simulink model "mazeSolving"  (R2023a)
settings: Solver=FixedStepDiscrete  StartTime=0.0  StopTime=120  FixedStep=0.01  RelTol=1e-3
values from neighbouring files (symbols this model uses):
  mapForSim =     [localisaton_obstacle_map.mat]
undefined symbols (not defined in the file or in its folder): axleLength, DiscIntNeverNeededParam, lineLength, wheelR
libraries: mobileRoboticsTrainingLib x2
settings Model: Creator=Boitumelo  LastModifiedBy=Nicola
settings DebuggingCC: UnconnectedInputMsg=warning  UnconnectedOutputMsg=warning  UnconnectedLineMsg=warning
settings ModelReferenceCC: EnableRefExpFcnMdlSchedulingChecks=on
settings RTWCC: DLArmComputeVersion=19.05

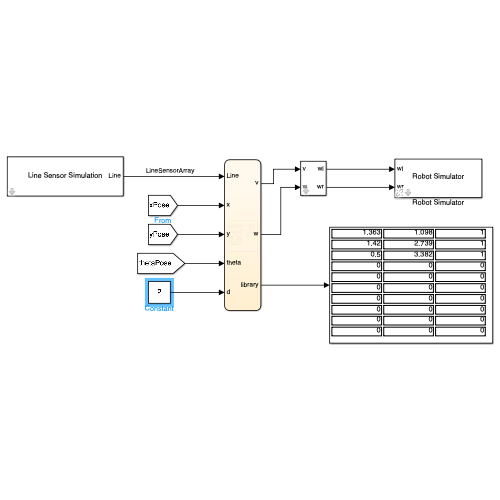
[thumbnail: Simulink's stored preview of the top-level diagram]
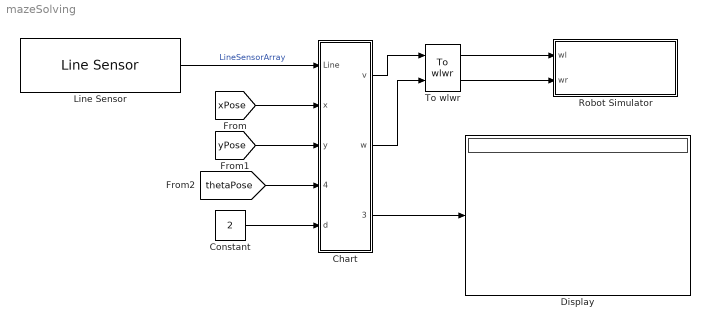
== system mazeSolving ==
  Chart : Stateflow chart  TreatAsAtomicUnit=on
      settings: PortSchema="{\"entries\":[{\"content\":{\"sides\":[{\"content\":{\"connectorIds\":[\"In1\",\"In2\",\"In3\",\"In4\",\"In5\"]},\"type\":\"ConnectorPlacement.EquallySpacedRectSide\",\"uuid\":\"117de8c6-9f64-465b-9576-500dc720da7e\"},{\"content\":{\"connectorIds\":[\"Out2\",\"Out1\",\"Out3\"],\"side\":\"RIGHT\"},\"type\":\"ConnectorPlacement.EquallySpacedRectSide\",\"uuid\":\"fddceec0-8182-4b0d-b09c-ad052d506c18\"},{\"content\":{\"side\":\"TOP\"},\"type\":\"ConnectorPlacement.EquallySpacedRectSide\",\"uuid\":\"0cbecf6e-5fd1-4495-a604-566e504879ee\"}]},\"type\":\"ConnectorPlacement.EquallySpacedConnector\",\"uuid\":\"83bd2747-f15a-41a4-a0f3-2474611a0dc7\"}],\"packageUris\":[\"http://schema.mathworks.com/mf0/Connector/R2020b\"],\"version\":\"1.0\"}"
  Constant : Constant  Value=2
  Display : Display
  Line Sensor : mobileRoboticsTrainingLib/Line Sensor  mapVariable=mapForSim  envVal=1  lineVal=0  sensOff=[0.0675 0.005; 0.0675 -0.005; 0.03 0.0354; 0.03 -0.0354]
      settings: SourceProductName=Mobile Robotics Training Library
  Robot Simulator : Subsystem  Priority=99  AncestorBlock=mobileRoboticsTrainingLib/Robot Simulator  mask(Robot Simulator){mapVar=mapForSim, startX=1.0088, startY=0.98472, startTheta=90, axleLength=axleLength, wheelR=wheelR}
      mask prompts: mapVar "Map Variable"; startX "Start X (m)"; startY "Start Y (m)"; startTheta "Theta (deg)"; axleLength "Axle Length (m)"; wheelR "Wheel Radius (m)"
      mask help: Configure robot simulator to use custom simulation maps and simulate closed-loop mobile robotics systems along with appropriate sensor simulation blocks.
      mask init:
      | set_param(bdroot,'SolverType','Fixed-Step');
      | set_param(bdroot,'Solver','FixedStepDiscrete');
      | 
      | if (exist('Ts'))
      |     set_param(bdroot,'FixedStep','Ts');
      | else
      |     set_param(bdroot,'FixedStep','0.01');
      | end
      | 
      | h = findobj('Name','Robot Simulator');
      | if ~isempty(h)
      |     close (h);
      | end
      | setupRobotSim();
      mask Help: web('Robot Simulator.htm')
      mask DialogControl mapCont Prompt: Map Setup
      mask DialogControl initPosCont Prompt: Initial Position
      mask DialogControl setPos Prompt: Set position interactively
      mask DialogControl setPos Callback:
      | %% Set starting point
      | setStartingPoint();
      mask DialogControl initOrientation Prompt: Initial Orientation
      mask DialogControl robotCharCont Prompt: Robot Characteristics
      mask Display: disp('Robot Simulator')
  To wlwr : mobileRoboticsTrainingLib/To wlwr  axleLength=axleLength  wheelR=wheelR
  wires:
  To wlwr/1 -> Robot Simulator/1(wl)
  To wlwr/2 -> Robot Simulator/2(wr)
  Line Sensor/1 -> Chart/1(Line)  "LineSensorArray"
  Chart/1(w) -> To wlwr/2
  Chart/2(v) -> To wlwr/1
  [xPose] -> Chart/2(x)
  [yPose] -> Chart/3(y)
  [thetaPose] -> Chart/4(theta)
  Chart/3(library) -> Display/1
  Constant/1 -> Chart/5(d)

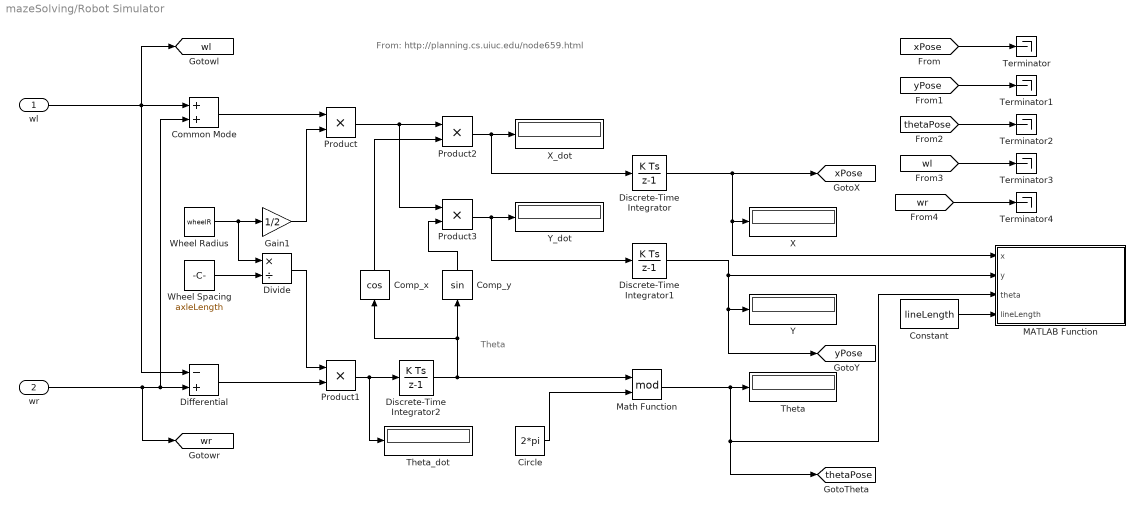
== system mazeSolving/Robot Simulator ==
  note: Theta
  note: From: http://planning.cs.uiuc.edu/node659.html
  wl : Inport
  wr : Inport  Port=2
  Circle : Constant  Value=2*pi
  Common Mode : Sum
  Comp_x : Trigonometry  Operator=cos
  Comp_y : Trigonometry
  Constant : Constant  Value=lineLength
  Differential : Sum  Inputs=-+
  Discrete-Time Integrator : DiscreteIntegrator  InitialCondition=startX  SampleTime=-1  ICPrevOutput=DiscIntNeverNeededParam  ICPrevScaledInput=DiscIntNeverNeededParam
  Discrete-Time Integrator1 : DiscreteIntegrator  InitialCondition=startY  SampleTime=-1  ICPrevOutput=DiscIntNeverNeededParam  ICPrevScaledInput=DiscIntNeverNeededParam
  Discrete-Time Integrator2 : DiscreteIntegrator  InitialCondition=startTheta*(pi/180)  SampleTime=-1  ICPrevOutput=DiscIntNeverNeededParam  ICPrevScaledInput=DiscIntNeverNeededParam
  Divide : Product  Inputs=*/
  Gain1 : Gain  Gain=1/2
  MATLAB Function : MATLAB Function  TreatAsAtomicUnit=on
  Math Function : Math  Operator=mod  SignedPower=on
  Product{,1..3} (4 alike) : Product  RndMeth=Zero
  Terminator{,1..4} (5 alike) : Terminator
  Theta : Display
  Theta_dot : Display
  Wheel Radius : Constant  Value=wheelR
  Wheel Spacing : Constant  Value=axleLength
  X : Display
  X_dot : Display
  Y : Display
  Y_dot : Display
  tag scope: thetaPose=global, wl=global, wr=global, xPose=global, yPose=global
  wires:
  [wr] -> Terminator4/1
  [wl] -> Terminator3/1
  Math Function/1 -> [thetaPose], MATLAB Function/3(theta), Theta/1
  Differential/1 -> Product1/2
  Comp_y/1 -> Product3/2
  Discrete-Time Integrator/1 -> [xPose], MATLAB Function/1(x), X/1
  Product3/1 -> Discrete-Time Integrator1/1, Y_dot/1
  Discrete-Time Integrator1/1 -> Y/1, [yPose], MATLAB Function/2(y)
  Divide/1 -> Product1/1
  wr/1 -> [wr], Common Mode/2, Differential/2
  Discrete-Time Integrator2/1 -> Math Function/1, Comp_x/1, Comp_y/1
  wl/1 -> [wl], Common Mode/1, Differential/1
  Comp_x/1 -> Product2/2
  Product1/1 -> Discrete-Time Integrator2/1, Theta_dot/1
  Wheel Radius/1 -> Divide/1, Gain1/1
  Wheel Spacing/1 -> Divide/2
  Product2/1 -> Discrete-Time Integrator/1, X_dot/1
  Gain1/1 -> Product/2
  Common Mode/1 -> Product/1
  Product/1 -> Product3/1, Product2/1
  Circle/1 -> Math Function/2
  Constant/1 -> MATLAB Function/4(lineLength)
  [xPose] -> Terminator/1
  [yPose] -> Terminator1/1
  [thetaPose] -> Terminator2/1

== matlab function mazeSolving/Robot Simulator/MATLAB Function ==
  data: x input; y input; theta input; lineLength input
function plotRobot(x,y,theta,lineLength)
% Get plot details
coder.extrinsic('evalin','plot')
ph1 = evalin('base','PlotHandle1');
ph2 = evalin('base','PlotHandle2');

% Find length orientation line
xp = [x x+lineLength*cos(theta)];
yp = [y y+lineLength*sin(theta)];

% Plot robot
set(ph1,'xdata',xp,'ydata',yp);
set(ph2,'xdata',x,'ydata',y);
drawnow('limitrate')

== stateflow chart mazeSolving/Chart ==
  state mazeSolving
    entry:
    n=1;
    library = zeros(10, 3);
    vDefault=0.2;
    branch=0;
    detect=0;
    during:
    L1 = Line(1);
    R1 = Line(2);
    L2 = Line(3);
    R2 = Line(4);
    state lineFollowing
      state goCW
        entry:
        w = -1;
        v=vDefault;
      state goStraight
        entry:
        w = 0;
        v=vDefault;
      state goCCW
        entry:
        w = 1;
        v=vDefault;
      (default) -> goStraight
      goCW -> goStraight : [L1==0]
      goCCW -> goStraight : [R1==0]
      goStraight -> goCW [order 2] : [L1==1]
      goStraight -> goCCW [order 1] : [R1==1]
    state detect
      entry:
      v=0;
      w=0;
      state measure
        entry:
        library(n, 1)=x;
        library(n, 2)=y;
        library(n,3)=d;
        n = n + 1;
        detect=1;
      (default) -> measure
    state turn180
      entry:
      theta0=theta;
      deltaTheta=abs(theta - theta0);
      during:
      v=0;
      w=-0.5;
      deltaTheta=abs(theta - theta0);
    state fork
      entry:
      fork=0;
      state startFork
        entry:
        v=0;
        w=0;
      state startBranch
        entry:
        branch=1;
        detect=0;
      state startMain
        entry:
        branch=0;
      state returnLeft
        during:
        v=0.02;
        w=0.5;
        exit:
        branchDirec=0;
      state turnRight1
        during:
        v=0.02;
        w=-0.5;
        exit:
        branchDirec=-0;
      state turnLeft
        during:
        v=0.02;
        w=0.5;
        exit:
        branchDirec=1;
      state turnRight
        during:
        v=0.02;
        w=-0.5;
        exit:
        branchDirec=-1;
      state endFork1
        entry:
        fork=1;
      (default) -> startFork
      startFork -> startBranch [order 1] : [branch==0]
      startFork -> startMain [order 2] : [branch==1]
      startMain -> returnLeft [order 1] : [branchDirec==1]
      startMain -> turnRight1 [order 2] : [branchDirec==-1]
      startBranch -> turnLeft [order 2] : [L2==0]
      startBranch -> turnRight [order 1] : [R2==0]
      returnLeft -> endFork1 : [theta>=1.5 && theta<3]
      turnRight1 -> endFork1 : [theta<=1.5]
      turnLeft -> endFork1 : [theta>=3]
      turnRight -> endFork1 : [theta>=6]
    state end
      entry:
      v=0;
      w=0;
    (default) -> lineFollowing
    lineFollowing -> detect [order 2] : [R1==1 && L1==1 && detect==0]
    detect -> turn180 : [detect==1]
    lineFollowing -> end [order 3] : [R1==0 && L1==0 && R2==0 && L2==0]
    turn180 -> lineFollowing : [deltaTheta>=3]
    lineFollowing -> fork [order 1] : [xor(R2==0, L2==0) || (R1==1 && L1==1 && detect==1)]
    fork -> lineFollowing : [fork==1]
  (default) -> mazeSolving
  data: w output; Line input; L2 local; R2 local; L1 local; R1 local; v output; vDefault local =0.02; x input; y input; n local; theta input; fork local; theta0 local; detect local; branch local; branchDirec local; deltaTheta local; library output; d input =1
